simulink model "Task4_1"  (R2020b)
settings: Solver=ode23t  StartTime=0.0  StopTime=10.0  RelTol=1e-3
values from neighbouring files (symbols this model uses):
  a1 = c0 * pi * rho * r^3    (= 10823.7684393)    [Code2021_Jo_Saleh.m]    (also in ExeRet21.m.m)
  a2 = c1 * pi * rho * r^4 / p    (= 2913.06360466)    [Code2021_Jo_Saleh.m]    (also in ExeRet21.m.m)
  a3 = 4 * c2 * pi * rho * r^5 / p^2    (= -341.490636632)    [Code2021_Jo_Saleh.m]    (also in ExeRet21.m.m)
  D = 0    [Code2021_Jo_Saleh.m]    (also in ExeRet21.m.m)
  dVw = 0.1    [Code2021_Jo_Saleh.m]    (also in ExeRet21.m.m)
  K = p * tau_z / (tau_pl * 2*we * tau_w)    (= -13.4008504823)    [Code2021_Jo_Saleh.m]    (also in ExeRet21.m.m)
  p = 180    [Code2021_Jo_Saleh.m]    (also in ExeRet21.m.m)
  Pel = Ptur    (= 3500000)    [Code2021_Jo_Saleh.m]    (also in ExeRet21.m.m)
  Pel_err = -50e3    (= -50000)    [Code2021_Jo_Saleh.m]    (also in ExeRet21.m.m)
  tau_i = 3e-3    (= 0.003)    [Code2021_Jo_Saleh.m]    (also in ExeRet21.m.m)
  tau_le = tau_w    (= 8.82652066845)    [Code2021_Jo_Saleh.m]    (also in ExeRet21.m.m)
  tau_lg = tau_z    (= -109.330180381)    [Code2021_Jo_Saleh.m]    (also in ExeRet21.m.m)
  tau_w = - 2 * J / (p * (a2*Vw_3 + a3*we_opt - D*2/p))    (= 8.82652066845)    [Code2021_Jo_Saleh.m]    (also in ExeRet21.m.m)
  tau_z = tau_w / (1 - p * tau_w * Te_opt / (2 * we_opt * J))    (= -109.330180381)    [Code2021_Jo_Saleh.m]    (also in ExeRet21.m.m)
  Te_rated = (Ptur * p) / (2 * we)    (= 1671126.90246)    [Code2021_Jo_Saleh.m]    (also in ExeRet21.m.m)
  Vw_3 = 10    [Code2021_Jo_Saleh.m]    (also in ExeRet21.m.m)
  we_opt = p / 2 * wm_opt    (= 120.6)    [Code2021_Jo_Saleh.m]    (also in ExeRet21.m.m)
settings Model: Creator=Tomo  LastModifiedBy=Tomo

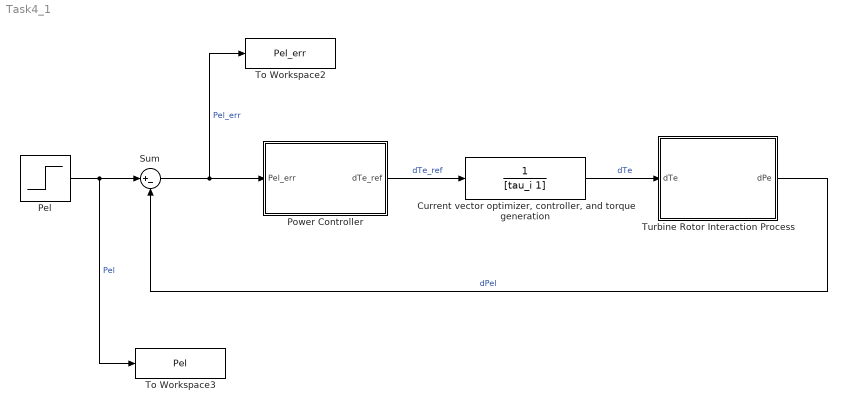
== system Task4_1 ==
  "Current vector optimizer, controller, and torque generation " : TransferFcn  Denominator=[tau_i 1]
  Pel : Step  Time=5  Before=Pel  After=Pel + Pel_err  SampleTime=0
  Power Controller : Subsystem
  Sum : Sum  Inputs=|+-
  To Workspace2 : ToWorkspace  VariableName=Pel_err  SampleTime=-1
  To Workspace3 : ToWorkspace  VariableName=Pel  SampleTime=-1
  Turbine Rotor Interaction Process : Subsystem
  wires:
  Sum/1 -> To Workspace2/1, Power Controller/1(Pel_err)  "Pel_err"
  Power Controller/1(dTe_ref) -> "Current vector optimizer, controller, and torque generation "/1  "dTe_ref"
  Turbine Rotor Interaction Process/1(dPe) -> Sum/2  "dPel"
  "Current vector optimizer, controller, and torque generation "/1 -> Turbine Rotor Interaction Process/1(dTe)  "dTe"
  Pel/1 -> Sum/1, To Workspace3/1  "Pel"

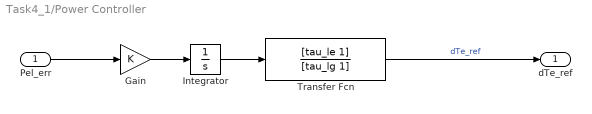
== system Task4_1/Power Controller ==
  Pel_err : Inport
  Gain : Gain  Gain=K
  Integrator : Integrator
  Transfer Fcn : TransferFcn  Numerator=[tau_le 1]  Denominator=[tau_lg 1]
  dTe_ref : Outport
  wires:
  Transfer Fcn/1 -> dTe_ref/1  "dTe_ref"
  Gain/1 -> Integrator/1
  Integrator/1 -> Transfer Fcn/1
  Pel_err/1 -> Gain/1

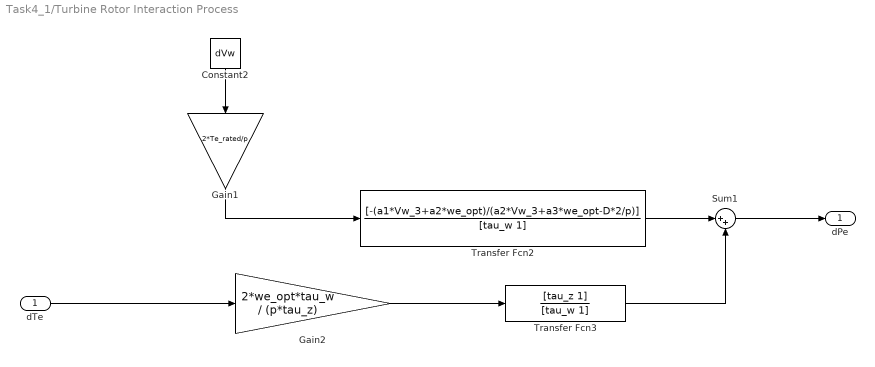
== system Task4_1/Turbine Rotor Interaction Process ==
  dTe : Inport
  Constant2 : Constant  Value=dVw
  Gain1 : Gain  Gain=2*Te_rated/p
  Gain2 : Gain  Gain=2*we_opt*tau_w / (p*tau_z)
  Sum1 : Sum  Inputs=|++
  Transfer Fcn2 : TransferFcn  Numerator=[-(a1*Vw_3+a2*we_opt)/(a2*Vw_3+a3*we_opt-D*2/p)]  Denominator=[tau_w 1]
  Transfer Fcn3 : TransferFcn  Numerator=[tau_z 1]  Denominator=[tau_w 1]
  dPe : Outport
  wires:
  Constant2/1 -> Gain1/1
  Sum1/1 -> dPe/1
  Transfer Fcn2/1 -> Sum1/1
  Gain2/1 -> Transfer Fcn3/1
  Transfer Fcn3/1 -> Sum1/2
  Gain1/1 -> Transfer Fcn2/1
  dTe/1 -> Gain2/1
